simulink model "untitled"  (R2024b)
settings: Solver=VariableStepAuto  StartTime=0.0  StopTime=10.0  RelTol=1e-3
settings Model: Creator=Berkay  LastModifiedBy=Berkay

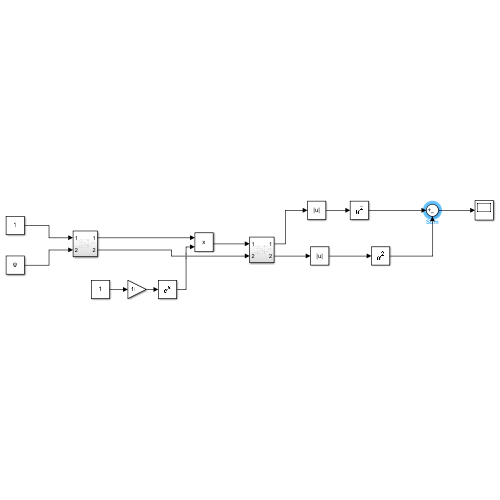
[thumbnail: Simulink's stored preview of the top-level diagram]
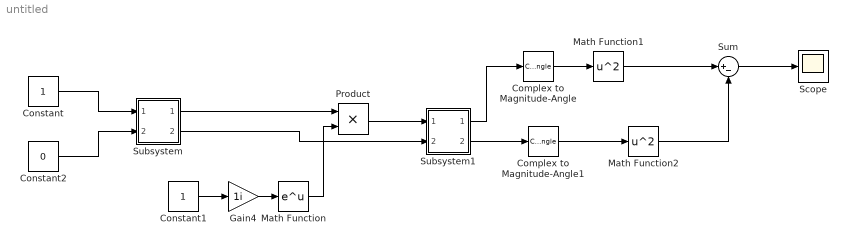
== system untitled ==
  Complex to Magnitude-Angle : ComplexToMagnitudeAngle  Output=Magnitude
  Complex to Magnitude-Angle1 : ComplexToMagnitudeAngle  Output=Magnitude
  Constant : Constant
  Constant1 : Constant
  Constant2 : Constant  Value=0
  Gain4 : Gain  Gain=1i
  Math Function : Math
  Math Function1 : Math  Operator=square
  Math Function2 : Math  Operator=square
  Product : Product
  Scope : Scope
  Subsystem : Subsystem
  Subsystem1 : Subsystem
  Sum : Sum  Inputs=|+-
  wires:
  Constant/1 -> Subsystem/1(In1)
  Constant2/1 -> Subsystem/2(In2)
  Subsystem/1(Out1) -> Product/1
  Subsystem/2(Out2) -> Subsystem1/2(In2)
  Subsystem1/2(Out2) -> Complex to Magnitude-Angle1/1
  Subsystem1/1(Out1) -> Complex to Magnitude-Angle/1
  Product/1 -> Subsystem1/1(In1)
  Gain4/1 -> Math Function/1
  Math Function/1 -> Product/2
  Constant1/1 -> Gain4/1
  Complex to Magnitude-Angle/1 -> Math Function1/1
  Complex to Magnitude-Angle1/1 -> Math Function2/1
  Math Function1/1 -> Sum/1
  Math Function2/1 -> Sum/2
  Sum/1 -> Scope/1

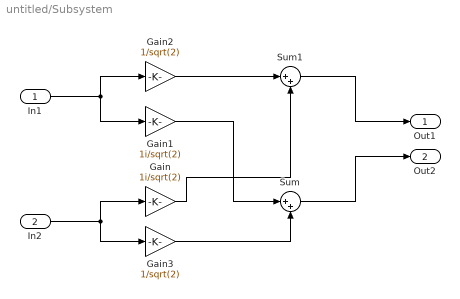
== system untitled/Subsystem ==
  In1 : Inport
  In2 : Inport  Port=2
  Gain : Gain  Gain=1i/sqrt(2)
  Gain1 : Gain  Gain=1i/sqrt(2)
  Gain2 : Gain  Gain=1/sqrt(2)
  Gain3 : Gain  Gain=1/sqrt(2)
  Sum : Sum  Inputs=|++
  Sum1 : Sum  Inputs=|++
  Out1 : Outport
  Out2 : Outport  Port=2
  wires:
  Gain2/1 -> Sum1/1
  Sum1/1 -> Out1/1
  In1/1 -> Gain1/1, Gain2/1
  Sum/1 -> Out2/1
  In2/1 -> Gain3/1, Gain/1
  Gain1/1 -> Sum/1
  Gain/1 -> Sum1/2
  Gain3/1 -> Sum/2

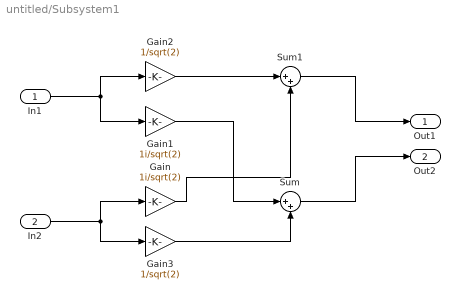
== system untitled/Subsystem1 ==
  In1 : Inport
  In2 : Inport  Port=2
  Gain : Gain  Gain=1i/sqrt(2)
  Gain1 : Gain  Gain=1i/sqrt(2)
  Gain2 : Gain  Gain=1/sqrt(2)
  Gain3 : Gain  Gain=1/sqrt(2)
  Sum : Sum  Inputs=|++
  Sum1 : Sum  Inputs=|++
  Out1 : Outport
  Out2 : Outport  Port=2
  wires:
  Gain2/1 -> Sum1/1
  Sum1/1 -> Out1/1
  In1/1 -> Gain1/1, Gain2/1
  Sum/1 -> Out2/1
  In2/1 -> Gain3/1, Gain/1
  Gain1/1 -> Sum/1
  Gain/1 -> Sum1/2
  Gain3/1 -> Sum/2
